simulink model "peltier_sim"  (R2024a)
settings: Solver=VariableStepAuto  StartTime=0.0  StopTime=100.0  RelTol=1e-3
libraries: cstblocks x1, slpidlib x1
settings Model: Creator=David  LastModifiedBy=David

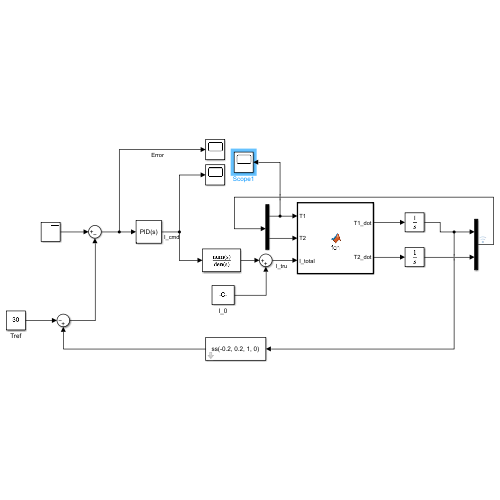
[thumbnail: Simulink's stored preview of the top-level diagram]
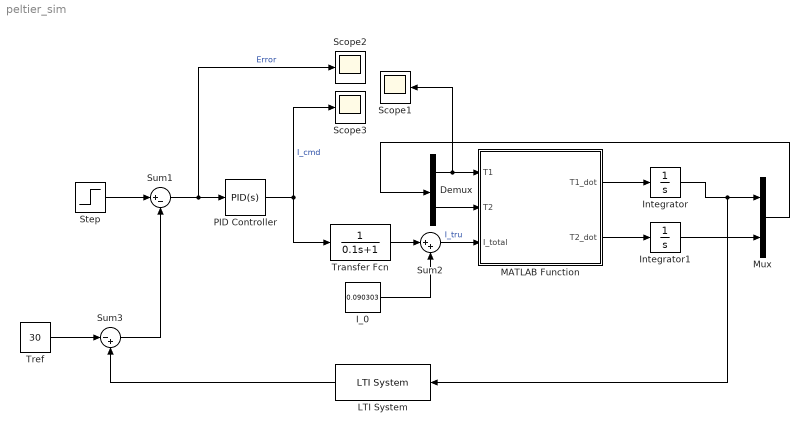
== system peltier_sim ==
  Demux : Demux  Outputs=2
  I_0 : Constant  Value=0.090303
  Integrator : Integrator  InitialCondition=30
  Integrator1 : Integrator  InitialCondition=23.1
  LTI System : cstblocks/LTI System  sys=ss(-0.2, 0.2, 1, 0)  IC=[30]  PadeOrder=0
  MATLAB Function : MATLAB Function  TreatAsAtomicUnit=on
  Mux : Mux  Inputs=2
  PID Controller : slpidlib/PID Controller  Controller=PID  Form=Parallel  TimeDomain=Continuous-time  UseExternalTs=off  SampleTime=-1  IntegratorMethod=Forward Euler  FilterMethod=Forward Euler  ControllerParametersSource=internal  P=0.352  I=0.005  UseKiTs=off  D=0.6  UseExternalDerivativeSource=off  N=0  UseFilter=on  TunerSelectOption=Transfer Function Based (PID Tuner App)  InitialConditionSource=internal  InitialConditionForIntegrator=0  InitialConditionForFilter=0  DifferentiatorICPrevScaledInput=0  ExternalReset=none  TrackingMode=off  Kt=1  LimitOutput=off  SatLimitsSource=internal  UpperSaturationLimit=inf  LowerSaturationLimit=-inf  LinearizeAsGain=on  AntiWindupMode=none  Kb=1  LimitIntegrator=off  UpperIntegratorSaturationLimit=inf  LowerIntegratorSaturationLimit=-inf  POutMin=[]  POutMax=[]  IOutMin=[]  IOutMax=[]  DOutMin=[]  DOutMax=[]  NOutMin=[]  NOutMax=[]  SumOutMin=[]  SumOutMax=[]  SaturationOutMin=[]  SaturationOutMax=[]  PParamMin=[]  PParamMax=[]  IParamMin=[]  IParamMax=[]  DParamMin=[]  DParamMax=[]  NParamMin=[]  NParamMax=[]  KbParamMin=[]  KbParamMax=[]  KtParamMin=[]  KtParamMax=[]  KbOutMin=[]  KbOutMax=[]  KtOutMin=[]  KtOutMax=[]  IntegratorOutMin=[]  IntegratorOutMax=[]  FilterOutMin=[]  FilterOutMax=[]  SumI1OutMin=[]  SumI1OutMax=[]  SumI2OutMin=[]  SumI2OutMax=[]  SumI3OutMin=[]  SumI3OutMax=[]  SumI4OutMin=[]  SumI4OutMax=[]  SumDOutMin=[]  SumDOutMax=[]  DifferentiatorOutMin=[]  DifferentiatorOutMax=[]  FilterDiffOutCoefMin=[]  FilterDiffOutCoefMax=[]  ReciprocalOutMin=[]  ReciprocalOutMax=[]  SumDenOutMin=[]  SumDenOutMax=[]  SumNumOutMin=[]  SumNumOutMax=[]  DivideOutMin=[]  DivideOutMax=[]  UdiffTsProdOutMin=[]  UdiffTsProdOutMax=[]  NTsProdOutMin=[]  NTsProdOutMax=[]  UintegralTsProdOutMin=[]  UintegralTsProdOutMax=[]  UngainTsProdOutMin=[]  UngainTsProdOutMax=[]  ClampingZeroOutDataTypeStr=Inherit: Inherit via back propagation  ClampingZeroOutMin=[]  ClampingZeroOutMax=[]  FilterDenConstantOutDataTypeStr=Inherit: Inherit via back propagation  FilterDenConstantOutMin=[]  FilterDenConstantOutMax=[]  PCopyOutDataTypeStr=Inherit: Inherit via back propagation  PCopyOutMin=[]  PCopyOutMax=[]  NCopyOutDataTypeStr=Inherit: Inherit via back propagation  NCopyOutMin=[]  NCopyOutMax=[]  IntegratorContinuousStateAttributes=''  IntegratorStateMustResolveToSignalObject=off  IntegratorRTWStateStorageClass=Auto  FilterContinuousStateAttributes=''  FilterStateMustResolveToSignalObject=off  FilterRTWStateStorageClass=Auto  ParallelPVariant=InternalParameters  IdealPVariant=Disabled  IVariant=InternalParameters  DVariant=InternalParameters  IntegratorVariant=Continuous  SatVariant=Disabled  AWVariant=Passthrough  PCopyVariant=Disabled  TRVariant=Disabled  FdbkBlocksVariant=Forward  IdealPFdbkVariant=Disabled  SatFdbkVariant=Disabled  DerivativeFilterVariant=ContFilter  NVariant=InternalParameters  NCopyVariant=Disabled  FilterICVariant=InternalICsFilter  IntegratorICVariant=InternalICs  ExternalResetVariant=Disabled  TRSumVariant=Passthrough  SumFdbkVariant=Disabled  SumVariant=Sum_PID  TsampFilterVariant=InternalTs  TsampNgainVariant=Passthrough  TsampIntegralVariant=Disabled_SignalSpec  ExternalSaturationOutDataTypeStr=Inherit: Same as second input  DerivativeSourceVariant=ErrorSignal
  Scope1 : Scope
  Scope2 : Scope
  Scope3 : Scope
  Step : Step  Time=0  SampleTime=0
  Sum1 : Sum  Inputs=|+-
  Sum2 : Sum  Inputs=|++
  Sum3 : Sum  Inputs=|-+
  Transfer Fcn : TransferFcn  Denominator=[0.1 1]
  Tref : Constant  Value=30
  wires:
  I_0/1 -> Sum2/2
  MATLAB Function/1(T1_dot) -> Integrator/1
  MATLAB Function/2(T2_dot) -> Integrator1/1
  Integrator1/1 -> Mux/2
  Demux/1 -> Scope1/1, MATLAB Function/1(T1)
  Demux/2 -> MATLAB Function/2(T2)
  Mux/1 -> Demux/1
  Sum1/1 -> Scope2/1, PID Controller/1  "Error"
  Step/1 -> Sum1/1
  Integrator/1 -> LTI System/1, Mux/1
  LTI System/1 -> Sum3/2
  Tref/1 -> Sum3/1
  Sum3/1 -> Sum1/2
  Transfer Fcn/1 -> Sum2/1
  PID Controller/1 -> Scope3/1, Transfer Fcn/1  "I_cmd"
  Sum2/1 -> MATLAB Function/3(I_total)  "I_tru"

== matlab function peltier_sim/MATLAB Function ==
  data: T1 input; T2 input; T1_dot output; I_total input; T2_dot output
function [T1_dot, T2_dot] = fcn(T1, T2, I_total)

    % Constants 
    n = 2.3279; C = 4.9013; K = 0.001255; G = 0.01279;
    R = 2.0000; alpha = 0.065036; Tinf = 24.3400;

    dT = T2 - T1;
    
    % Use (:) or index explicitly if T1/T2 are coming in as vectors
    T1_dot = (1/C) * ( K*sign(dT)*abs(dT)^n + 0.5*R*I_total^2 + alpha*I_total*T1 + G*(Tinf - T1));
    T2_dot = (1/C) * (-K*sign(dT)*abs(dT)^n + 0.5*R*I_total^2 - alpha*I_total*T2 + G*(Tinf - T2));
end
